simulink library "SUB_L4_Task_10000ms"  (R2018a)
settings: Solver=VariableStepAuto  StartTime=0.0  StopTime=10.0  RelTol=1e-3
libraries: simulink x1
settings Model: Creator=Chris.Balton  LastModifiedBy=Chris.Balton

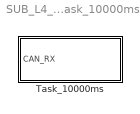
== system SUB_L4_Task_10000ms ==
  Task_10000ms : Subsystem  TreatAsAtomicUnit=on  SystemSampleTime=10

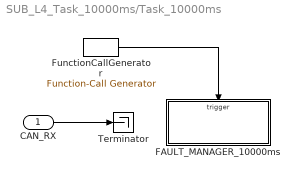
== system SUB_L4_Task_10000ms/Task_10000ms ==
  CAN_RX : Inport
  FAULT_MANAGER_10000ms : Subsystem
  FunctionCallGenerator : simulink/Ports & Subsystems/Function-Call Generator  sample_time=-1  numberOfIterations=1
  Terminator : Terminator
  wires:
  CAN_RX/1 -> Terminator/1
  FunctionCallGenerator/1 -> FAULT_MANAGER_10000ms/Trigger

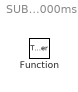
== system SUB_L4_Task_10000ms/Task_10000ms/FAULT_MANAGER_10000ms ==
  Function : TriggerPort  TriggerType=function-call  VariantControl=(inherit)
      settings: AttributesFormatString=States when enabling: %<StatesWhenEnabling>
